simulink model "Mpc_RealTime_with_standing"  (R2017b)
settings: Solver=FixedStepDiscrete  StartTime=0.0  StopTime=inf  FixedStep=0.0005  RelTol=1e-3  EnableMultiTasking=on
InitFcn:
  | isSim = 0;
  | PreFunctions.CustomInitFcn_with_standing;
undefined symbols (not defined in the file): DynamicMatrixLibrary, sample_time
libraries: slrtlib x29, xpcrtudplib x2, xpcutilitieslib x1, CassieLibrary x1
settings Model: xpc_rtwmakecfg_data=_xpcethercatlib_  TunableVars=c_CovPos_abduction,c_CovPos_knee,c_CovPos_qj1,c_CovPos_qj2,c_CovPos_qj3,c_CovPos_rotation,c_CovPos_thigh,c_CovPos_toe,c_CovVel_abduction,c_CovVel_knee,c_CovVel_qj1,c_CovVel_qj2,c_CovVel_qj3,c_CovVel_rotation,c_CovVel_thigh,c_CovVel_toe,c_Cov_AngularVelocity,c_Cov_Euler,c_Cov_Euler_rates,c_Cov_LinearAccelerator_xy,c_Cov_LinearAccelerator_z,c_Cov_Lx_LRToe_stTD0,c_Cov_Ly_LRToe_stTD0,c_Cov_Orientation,c_Cov_rpx_LRToe_body,c_Cov_rpx_LRToe_stTD0,c_Cov_rpy_LRToe_body,c_Cov_rpy_LRToe_stTD0,c_Cov_rpz_LRToe_body,c_H_fil_param,c_IK_max_iter_num,c_Kd_abduction,c_Kd_knee,c_Kd_pitch,c_Kd_roll,c_Kd_rotation,c_Kd_st_rotation,c_Kd_thigh,c_Kd_toe,c_Kd_yaw,c_Kp_abduction,c_Kp_knee,c_Kp_pitch,c_Kp_roll,c_Kp_rotation,c_Kp_st_rotation,c_Kp_thigh,c_Kp_toe,c_Kp_yaw,c_KsL_1,c_KsL_2,c_KsR_1,c_KsR_2,c_Tx_slide_toe_2,c_Ty_slide_toe_2,c_Tz_slide_toe_2,c_Vx_tgd_fil_param,c_Vx_tgd_offset,c_Vy_tgd_avg_fil_param,c_Vy_tgd_offset,c_adjusted_desired_roll_angle_fil_param,c_com_x_offset,c_desired_com2stToe_lateral_fil_param,c_dop,c_history_length,c_knee_cp_time,c_lateral_correction_gain,c_max_st_rotation_motor_torque,c_max_turn_per_sec,c_one_step_max_vel_gain,c_rp_LRToe_fil_param,c_st_rotation_torque_ramp_time,c_stance_thre_lb,c_stance_thre_lb_2,c_stance_thre_ub,c_stance_thre_ub_2,c_toe_leave_ground_lb,c_toe_leave_ground_ub,c_torque_transition_time,c_u_abduction_swing_cp,c_u_knee_cp,c_u_pitch_cp,c_u_roll_cp,c_use_dq_AR_for_PD,c_vx_slide_toe_1,c_vx_slide_toe_2,c_vy_slide_toe_1,c_vy_slide_toe_2,c_vz_slide_toe_1,c_vz_slide_toe_2,c_yaw_error_fil_param  TunableVarsStorageClass=Auto,Auto,Auto,Auto,Auto,Auto,Auto,Auto,Auto,Auto,Auto,Auto,Auto,Auto,Auto,Auto,Auto,Auto,Auto,Auto,Auto,Auto,Auto,Auto,Auto,Auto,Auto,Auto,Auto,Auto,Auto,Auto,Auto,Auto,Auto,Auto,Auto,Auto,Auto,Auto,Auto,Auto,Auto,Auto,Auto,Auto,Auto,Auto,Auto,Auto,Auto,Auto,Auto,Auto,Auto,Auto,Auto,Auto,Auto,Auto,Auto,Auto,Auto,Auto,Auto,Auto,Auto,Auto,Auto,Auto,Auto,Auto,Auto,Auto,Auto,Auto,Auto,Auto,Auto,Auto,Auto,Auto,Auto,Auto,Auto,Auto,Auto,Auto,Auto,Auto,Auto  TunableVarsTypeQualifier=,,,,,,,,,,,,,,,,,,,,,,,,,,,,,,,,,,,,,,,,,,,,,,,,,,,,,,,,,,,,,,,,,,,,,,,,,,,,,,,,,,,,,,,,,,  Creator=robot  LastModifiedBy=gibso
settings DataIOCC: SaveFormat=Array  SaveOutput=off  SignalLogging=off  DSMLogging=off  VisualizeSimOutput=off  SaveTime=off
settings OptimizationCC: LifeSpan=inf  SimCompilerOptimization=on  AccelVerboseBuild=on
settings DebuggingCC: AllowSymbolicDim=off  SFUnexpectedBacktrackingDiag=warning  SFNoUnconditionalDefaultTransitionDiag=warning  SFExecutionAtInitializationDiag=none
settings HardwareCC: ProdBitPerPointer=32  ProdBitPerSizeT=32  ProdBitPerPtrDiffT=32  ProdLargestAtomicFloat=None  ProdWordSize=32  ProdLongLongMode=on  ProdHWDeviceType=Generic->32-bit x86 compatible
settings ModelReferenceCC: ParallelModelReferenceMATLABWorkerInit=Copy Base Workspace  ModelReferenceNumInstancesAllowed=Zero  PropagateSignalLabelsOutOfModel=off
settings SFSimCC: SimUserIncludeDirs=C:\Users\gibso\workspace\research\cassie_mpc_lip\matlab\Custom_Code\utils\funcs\KinDyn200511_221619  SFSimEcho=off
settings SFSimCC: SimUserSources=|
  | R_LeftAbductionJoint_src.c
  | R_LeftThighJoint_src.c
  | R_RightAbductionJoint_src.c
  | R_RightThighJoint_src.c
  | 
  | AMworld_about_pA_src.c
  | 
  | Jb_BasePosX_src.c
  | Jb_BasePosY_src.c
  | Jb_BasePosZ_src.c
  | Jb_BaseRotX_src.c
  | Jb_BaseRotY_src.c
  | Jb_BaseRotZ_src.c
  | Jb_LeftAbductionJoint_src.c
  | Jb_LeftAnkleJoint_src.c
  | Jb_LeftHip_src.c
  | Jb_LeftKneeJoint_src.c
  | Jb_LeftKneeSpringJoint_src.c
  | Jb_LeftKnee_src.c
  | Jb_LeftPelvisRotation_src.c
  | Jb_LeftRotationJoint_src.c
  | Jb_LeftShin_src.c
  | Jb_LeftTarsus_src.c
  | Jb_LeftThighJoint_src.c
  | Jb_LeftThigh_src.c
  | Jb_LeftToeBottomBack_src.c
  | Jb_LeftToeBottomFront_src.c
  | Jb_LeftToeBottom_src.c
  | Jb_LeftToeJoint_src.c
  | Jb_LeftToe_src.c
  | Jb_Pelvis_src.c
  | Jb_RightAbductionJoint_src.c
  | Jb_RightAnkleJoint_src.c
  | Jb_RightHip_src.c
  | Jb_RightKneeJoint_src.c
  | Jb_RightKneeSpringJoint_src.c
  | Jb_RightKnee_src.c
  | Jb_RightPelvisRotation_src.c
  | Jb_RightRotationJoint_src.c
  | Jb_RightShin_src.c
  | Jb_RightTarsus_src.c
  | Jb_RightThighJoint_src.c
  | Jb_RightThigh_src.c
  | Jb_RightToeBottomBack_src.c
  | Jb_RightToeBottomFront_src.c
  | Jb_RightToeBottom_src.c
  | Jb_RightToeJoint_src.c
  | Jb_RightToe_src.c
  | 
  | Jdq_AMworld_about_pA_src.c
  | 
  | 
  | Jp_COM_src.c
  | Jp_LeftAbductionJoint_src.c
  | Jp_LeftAnkleJoint_src.c
  | Jp_LeftHip_src.c
  | Jp_LeftKneeJoint_src.c
  | Jp_LeftKneeSpringJoint_src.c
  | Jp_LeftKnee_src.c
  | Jp_LeftPelvisRotation_src.c
  | Jp_LeftRotationJoint_src.c
  | Jp_LeftShin_src.c
  | Jp_LeftTarsus_src.c
  | Jp_LeftThighJoint_src.c
  | Jp_LeftThigh_src.c
  | Jp_LeftToeBottomBack_src.c
  | Jp_LeftToeBottomFront_src.c
  | Jp_LeftToeBottom_src.c
  | Jp_LeftToeJoint_src.c
  | Jp_LeftToe_src.c
  | Jp_Pelvis_src.c
  | Jp_RightAbductionJoint_src.c
  | Jp_RightAnkleJoint_src.c
  | Jp_RightHip_src.c
  | Jp_RightKneeJoint_src.c
  | Jp_RightKneeSpringJoint_src.c
  | Jp_RightKnee_src.c
  | Jp_RightPelvisRotation_src.c
  | Jp_RightRotationJoint_src.c
  | Jp_RightShin_src.c
  | Jp_RightTarsus_src.c
  | Jp_RightThighJoint_src.c
  | Jp_RightThigh_src.c
  | Jp_RightToeBottomBack_src.c
  | Jp_RightToeBottomFront_src.c
  | Jp_RightToeBottom_src.c
  | Jp_RightToeJoint_src.c
  | Jp_RightToe_src.c
  | 
  | p_BasePosX_src.c
  | p_BasePosY_src.c
  | p_BasePosZ_src.c
  | p_BaseRotX_src.c
  | p_BaseRotY_src.c
  | p_BaseRotZ_src.c
  | p_COM_src.c
  | p_LeftAbductionJoint_src.c
  | p_LeftAnkleJoint_src.c
  | p_LeftHip_src.c
  | p_LeftKneeJoint_src.c
  | p_LeftKneeSpringJoint_src.c
  | p_LeftKnee_src.c
  | p_LeftPelvisRotation_src.c
  | p_LeftRotationJoint_src.c
  | p_LeftShin_src.c
  | p_LeftTarsus_src.c
  | p_LeftThighJoint_src.c
  | p_LeftThigh_src.c
  | p_LeftToeBottomBack_src.c
  | p_LeftToeBottomFront_src.c
  | p_LeftToeBottom_src.c
  | p_LeftToeJoint_src.c
  | p_LeftToe_src.c
  | p_Pelvis_src.c
  | p_RightAbductionJoint_src.c
  | p_RightAnkleJoint_src.c
  | p_RightHip_src.c
  | p_RightKneeJoint_src.c
  | p_RightKneeSpringJoint_src.c
  | p_RightKnee_src.c
  | p_RightPelvisRotation_src.c
  | p_RightRotationJoint_src.c
  | p_RightShin_src.c
  | p_RightTarsus_src.c
  | p_RightThighJoint_src.c
  | p_RightThigh_src.c
  | p_RightToeBottomBack_src.c
  | p_RightToeBottomFront_src.c
  | p_RightToeBottom_src.c
  | p_RightToeJoint_src.c
  | p_RightToe_src.c
  | 
  | T_LeftToeBottomBack_src.c
  | T_LeftToeBottomFront_src.c
  | T_LeftToeBottom_src.c
  | T_RightToeBottomBack_src.c
  | T_RightToeBottomFront_src.c
  | T_RightToeBottom_src.c
  | 
  | J_LL_Left_src.c
  | J_LL_Right_src.c
  | LL_Left_src.c
  | LL_Right_src.c
settings RTWCC: SystemTargetFile=slrt.tlc  TLCOptions=-axPCMaxOverloads=1000000000 -axPCMaxOverloadLen=1000000000  TemplateMakefile=slrt_default_tmf  Description=Simulink Real-Time  RTWUseSimCustomCode=on  CustomInclude=C:\Users\gibso\workspace\research\cassie_mpc_lip\matlab\Custom_Code\utils\funcs\KinDyn200511_221619  CodeExecutionProfiling=on  RTWCompilerOptimization=on
settings RTWCC: CustomSource=|
  | R_LeftAbductionJoint_src.c
  | R_LeftThighJoint_src.c
  | R_RightAbductionJoint_src.c
  | R_RightThighJoint_src.c
  | 
  | AMworld_about_pA_src.c
  | 
  | Jb_BasePosX_src.c
  | Jb_BasePosY_src.c
  | Jb_BasePosZ_src.c
  | Jb_BaseRotX_src.c
  | Jb_BaseRotY_src.c
  | Jb_BaseRotZ_src.c
  | Jb_LeftAbductionJoint_src.c
  | Jb_LeftAnkleJoint_src.c
  | Jb_LeftHip_src.c
  | Jb_LeftKneeJoint_src.c
  | Jb_LeftKneeSpringJoint_src.c
  | Jb_LeftKnee_src.c
  | Jb_LeftPelvisRotation_src.c
  | Jb_LeftRotationJoint_src.c
  | Jb_LeftShin_src.c
  | Jb_LeftTarsus_src.c
  | Jb_LeftThighJoint_src.c
  | Jb_LeftThigh_src.c
  | Jb_LeftToeBottomBack_src.c
  | Jb_LeftToeBottomFront_src.c
  | Jb_LeftToeBottom_src.c
  | Jb_LeftToeJoint_src.c
  | Jb_LeftToe_src.c
  | Jb_Pelvis_src.c
  | Jb_RightAbductionJoint_src.c
  | Jb_RightAnkleJoint_src.c
  | Jb_RightHip_src.c
  | Jb_RightKneeJoint_src.c
  | Jb_RightKneeSpringJoint_src.c
  | Jb_RightKnee_src.c
  | Jb_RightPelvisRotation_src.c
  | Jb_RightRotationJoint_src.c
  | Jb_RightShin_src.c
  | Jb_RightTarsus_src.c
  | Jb_RightThighJoint_src.c
  | Jb_RightThigh_src.c
  | Jb_RightToeBottomBack_src.c
  | Jb_RightToeBottomFront_src.c
  | Jb_RightToeBottom_src.c
  | Jb_RightToeJoint_src.c
  | Jb_RightToe_src.c
  | 
  | Jdq_AMworld_about_pA_src.c
  | 
  | 
  | Jp_COM_src.c
  | Jp_LeftAbductionJoint_src.c
  | Jp_LeftAnkleJoint_src.c
  | Jp_LeftHip_src.c
  | Jp_LeftKneeJoint_src.c
  | Jp_LeftKneeSpringJoint_src.c
  | Jp_LeftKnee_src.c
  | Jp_LeftPelvisRotation_src.c
  | Jp_LeftRotationJoint_src.c
  | Jp_LeftShin_src.c
  | Jp_LeftTarsus_src.c
  | Jp_LeftThighJoint_src.c
  | Jp_LeftThigh_src.c
  | Jp_LeftToeBottomBack_src.c
  | Jp_LeftToeBottomFront_src.c
  | Jp_LeftToeBottom_src.c
  | Jp_LeftToeJoint_src.c
  | Jp_LeftToe_src.c
  | Jp_Pelvis_src.c
  | Jp_RightAbductionJoint_src.c
  | Jp_RightAnkleJoint_src.c
  | Jp_RightHip_src.c
  | Jp_RightKneeJoint_src.c
  | Jp_RightKneeSpringJoint_src.c
  | Jp_RightKnee_src.c
  | Jp_RightPelvisRotation_src.c
  | Jp_RightRotationJoint_src.c
  | Jp_RightShin_src.c
  | Jp_RightTarsus_src.c
  | Jp_RightThighJoint_src.c
  | Jp_RightThigh_src.c
  | Jp_RightToeBottomBack_src.c
  | Jp_RightToeBottomFront_src.c
  | Jp_RightToeBottom_src.c
  | Jp_RightToeJoint_src.c
  | Jp_RightToe_src.c
  | 
  | p_BasePosX_src.c
  | p_BasePosY_src.c
  | p_BasePosZ_src.c
  | p_BaseRotX_src.c
  | p_BaseRotY_src.c
  | p_BaseRotZ_src.c
  | p_COM_src.c
  | p_LeftAbductionJoint_src.c
  | p_LeftAnkleJoint_src.c
  | p_LeftHip_src.c
  | p_LeftKneeJoint_src.c
  | p_LeftKneeSpringJoint_src.c
  | p_LeftKnee_src.c
  | p_LeftPelvisRotation_src.c
  | p_LeftRotationJoint_src.c
  | p_LeftShin_src.c
  | p_LeftTarsus_src.c
  | p_LeftThighJoint_src.c
  | p_LeftThigh_src.c
  | p_LeftToeBottomBack_src.c
  | p_LeftToeBottomFront_src.c
  | p_LeftToeBottom_src.c
  | p_LeftToeJoint_src.c
  | p_LeftToe_src.c
  | p_Pelvis_src.c
  | p_RightAbductionJoint_src.c
  | p_RightAnkleJoint_src.c
  | p_RightHip_src.c
  | p_RightKneeJoint_src.c
  | p_RightKneeSpringJoint_src.c
  | p_RightKnee_src.c
  | p_RightPelvisRotation_src.c
  | p_RightRotationJoint_src.c
  | p_RightShin_src.c
  | p_RightTarsus_src.c
  | p_RightThighJoint_src.c
  | p_RightThigh_src.c
  | p_RightToeBottomBack_src.c
  | p_RightToeBottomFront_src.c
  | p_RightToeBottom_src.c
  | p_RightToeJoint_src.c
  | p_RightToe_src.c
  | 
  | T_LeftToeBottomBack_src.c
  | T_LeftToeBottomFront_src.c
  | T_LeftToeBottom_src.c
  | T_RightToeBottomBack_src.c
  | T_RightToeBottomFront_src.c
  | T_RightToeBottom_src.c
  | 
  | J_LL_Left_src.c
  | J_LL_Right_src.c
  | LL_Left_src.c
  | LL_Right_src.c
settings CodeAppCC: GenerateComments=off  MaxIdLength=128  SimulinkBlockComments=off
settings ConfigComp: CovMetricSettings=dw  CovHtmlReporting=on  CovSaveCumulativeToWorkspaceVar=on  CovSaveSingleToWorkspaceVar=on  CovExternalEMLEnable=off

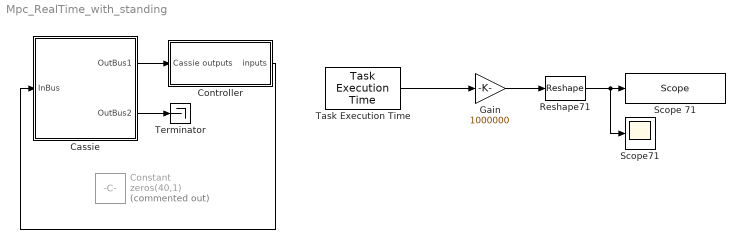
== system Mpc_RealTime_with_standing ==
  Cassie : Subsystem  AncestorBlock=CassieLibrary/RealTime/Cassie  InitFcn=|
      | % Import bus definitions
      | CassieModule.importBuses;
      mask Display: image('Cassie.png');
  Constant : Constant  Commented=on  Value=zeros(40,1)
  Controller : Subsystem
  Gain : Gain  Gain=1000000
  Reshape71 : Reshape
  Scope 71 : slrtlib/Displays and Logging/Scope   scopeno=1234  scopetype=Host  autostart=on  viewmode=Graphical redraw  formatstr='%15.6f'  grid=on  ylimits=[0,0]  nosamples=2500  noprepostsamples=0  interleave=1  triggermode=FreeRun  triggersignal=1  trigsignalfromport=off  triggerlevel=0.0  triggerslope=Either  triggerscope=1  triggersample=0  filename=data.dat  mode=Lazy  writesize=512  autorestart=off  dynamicfilemode=off  maxwritefilesize=512*1024^2
  Scope71 : Scope
  "Task Execution Time " : slrtlib/Target Management/Execution Parameters/Task Execution Time   ts=0.0005
      settings: SourceProductName=Simulink Real-Time  SourceProductBaseCode=XP
  Terminator : Terminator
  wires:
  Controller/1("inputs ") -> Cassie/1(InBus)
  Cassie/1(OutBus1) -> Controller/1(Cassie outputs)
  Reshape71/1 -> Scope71/1, Scope 71/1
  "Task Execution Time "/1 -> Gain/1
  Gain/1 -> Reshape71/1
  Cassie/2(OutBus2) -> Terminator/1

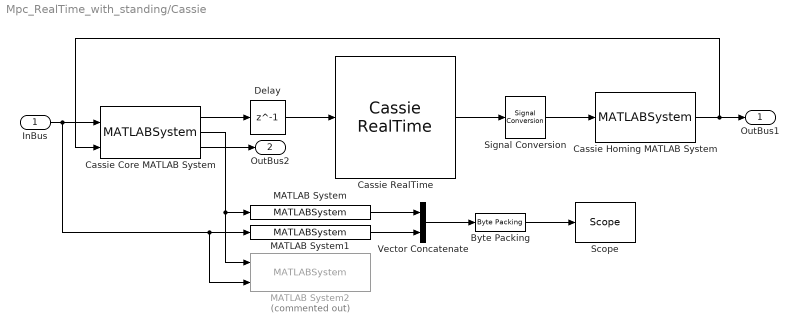
== system Mpc_RealTime_with_standing/Cassie ==
  InBus : Inport  OutDataTypeStr=Bus: CassieUserInBus
  "Byte Packing " : xpcutilitieslib/Byte Packing   MaskPackedDataType=double  MaskUnpackedDataTypes={'uint8'}  MaskAlignment=1
  Cassie Core MATLAB System : MATLABSystem  System=CassieCore  SimulateUsing=Code generation
      mask Type: CassieCore
      mask Display: disp('CassieCore');
  Cassie Homing MATLAB System : MATLABSystem  System=CassieHoming  SimulateUsing=Code generation
      mask Type: CassieHoming
      mask Display: disp('CassieHoming');
  Cassie RealTime : CassieLibrary/RealTime/Cassie RealTime  SystemSampleTime=-1
  Delay : Delay  DelayLength=1
  MATLAB System : MATLABSystem  System=CassieOutBusToBytes  SimulateUsing=Code generation
      mask Type: CassieOutBusToBytes
      mask Display: disp('CassieOutBusToBytes');
  MATLAB System1 : MATLABSystem  System=CassieUserInBusToBytes  SimulateUsing=Code generation
      mask Type: CassieUserInBusToBytes
      mask Display: disp('CassieUserInBusToBytes');
  MATLAB System2 : MATLABSystem  Commented=on  System=CassieSummaryLogger  period=1000  SimulateUsing=Code generation
      mask Type: CassieSummaryLogger
      mask Display: disp('CassieSummaryLogger');
  "Scope " : slrtlib/Displays and Logging/Scope   scopeno=1  scopetype=File  autostart=on  viewmode=Graphical redraw  formatstr='%15.6f'  grid=on  ylimits=[0,0]  nosamples=250  noprepostsamples=0  interleave=1  triggermode=FreeRun  triggersignal=1  trigsignalfromport=off  triggerlevel=0.0  triggerslope=Either  triggerscope=1  triggersample=0  filename=cassie<%%>.dat  mode=Commit  writesize=4096  autorestart=on  dynamicfilemode=on  maxwritefilesize=1024^3
  Signal Conversion : SignalConversion  ConversionOutput=Nonvirtual bus  OutDataTypeStr=Bus: CassieOutBus  OverrideOpt=off
  Vector Concatenate : Concatenate
  OutBus1 : Outport  OutDataTypeStr=Bus: CassieOutBus
  OutBus2 : Outport  Port=2  OutDataTypeStr=boolean
  wires:
  Cassie Core MATLAB System/3 -> OutBus2/1
  Cassie Core MATLAB System/2 -> MATLAB System/1, MATLAB System2/1
  "Byte Packing "/1 -> "Scope "/1
  MATLAB System1/1 -> Vector Concatenate/2
  Vector Concatenate/1 -> "Byte Packing "/1
  MATLAB System/1 -> Vector Concatenate/1
  Cassie Homing MATLAB System/1 -> OutBus1/1, Cassie Core MATLAB System/2
  Signal Conversion/1 -> Cassie Homing MATLAB System/1
  Delay/1 -> Cassie RealTime/1
  Cassie Core MATLAB System/1 -> Delay/1
  InBus/1 -> MATLAB System1/1, MATLAB System2/2, Cassie Core MATLAB System/1
  Cassie RealTime/1 -> Signal Conversion/1

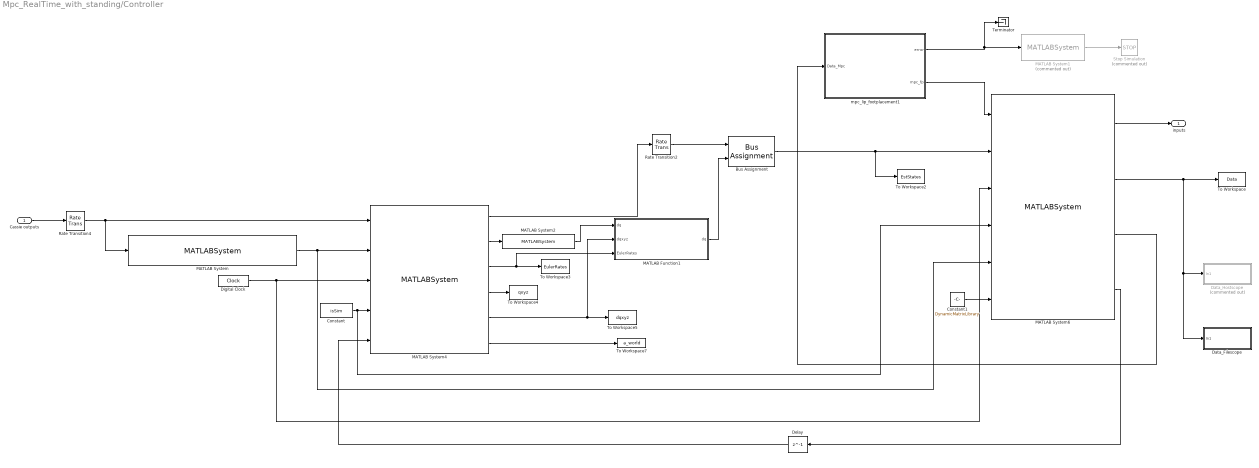
== system Mpc_RealTime_with_standing/Controller ==
  Cassie outputs : Inport  OutDataTypeStr=Bus: CassieOutBus
  Bus Assignment : BusAssignment  AssignedSignals=dq
  Constant : Constant  Value=isSim  OutDataTypeStr=int8  LockScale=on
  Constant1 : Constant  Value=DynamicMatrixLibrary  OutDataTypeStr=Bus: cassieDynamicMatrixLibraryBus
  Data_Filescope : Subsystem
  Data_Hostscope : Subsystem  Commented=on
  Delay : Delay  DelayLength=1  InitialCondition=0
  Digital Clock : DigitalClock  SampleTime=sample_time
  MATLAB Function1 : MATLAB Function  TreatAsAtomicUnit=on
  MATLAB System : MATLABSystem  System=RadioCommandInterpreter_with_standing  max_turn_per_sec=c_max_turn_per_sec  Vx_tgd_fil_param=c_Vx_tgd_fil_param  Vy_tgd_avg_fil_param=c_Vy_tgd_avg_fil_param  H_fil_param=c_H_fil_param  desired_com2stToe_lateral_fil_param=c_desired_com2stToe_lateral_fil_param  yaw_stand_filter_param=c_yaw_stand_filter_param  pitch_stand_filter_param=c_pitch_stand_filter_param  roll_stand_filter_param=c_roll_stand_filter_param  p_com_stand_y_filter_param=c_p_com_stand_y_filter_param  sample_time=sample_time  SimulateUsing=Code generation
      mask Type: RadioCommandInterpreter_with_standing
      mask Display:
      | disp('RadioCommandInterpreter_with_standing');
      | port_label('input',1,'cassieOutputs');
      | port_label('output',1,'IRC');
  MATLAB System1 : MATLABSystem  Commented=on  System=Error_Checker  SimulateUsing=Code generation
      mask Type: Error_Checker
      mask Display:
      | disp('Error_Checker');
      | port_label('input',1,'u');
      | port_label('output',1,'y');
  MATLAB System2 : MATLABSystem  System=PolyRegressionFilter_2  sample_time=sample_time  history_length=c_history_length  dop=c_dop  signal_dim=20  delay=0  max_history_length=20  max_dop=3  SimulateUsing=Code generation
      mask Type: PolyRegressionFilter_2
      mask Display:
      | disp('PolyRegressionFilter_2');
      | port_label('input',1,'q');
      | port_label('output',1,'dq');
  MATLAB System4 : MATLABSystem  System=StateEstimator_with_standing  Ks_L1=c_KsL_1  Ks_L2=c_KsL_2  Ks_R1=c_KsR_1  Ks_R2=c_KsR_2  Cov_LRT_r_body_x=c_Cov_rpx_LRToe_body  Cov_LRT_r_body_y=c_Cov_rpy_LRToe_body  Cov_LRT_r_body_z=c_Cov_rpz_LRToe_body  Cov_LinearAccelerator_xy=c_Cov_LinearAccelerator_xy  Cov_LinearAccelerator_z=c_Cov_LinearAccelerator_z  vx_slide_toe_1=c_vx_slide_toe_1  vx_slide_toe_2=c_vx_slide_toe_2  Tx_slide_toe_2=c_Tx_slide_toe_2  vy_slide_toe_1=c_vy_slide_toe_1  vy_slide_toe_2=c_vy_slide_toe_2  Ty_slide_toe_2=c_Ty_slide_toe_2  vz_slide_toe_1=c_vz_slide_toe_1  vz_slide_toe_2=c_vz_slide_toe_2  Tz_slide_toe_2=c_Tz_slide_toe_2  sample_time=sample_time  SimulateUsing=Code generation
      mask Type: StateEstimator_with_standing
      mask Display:
      | disp('StateEstimator_with_standing');
      | port_label('input',1,'cassieOutputs');
      | port_label('input',2,'IRC');
      | port_label('input',3,'t_total');
      | port_label('input',4,'isSim');
      | port_label('input',5,'Controller2Estimator');
      | port_label('output',1,'EstStates');
      | port_label('output',2,'q');
      | port_label('output',3,'EulerRates');
      | port_label('output',4,'q_xyz');
      | port_label('output',5,'dq_xyz');
      | port_label('output',6,'a_world');
  MATLAB System6 : MATLABSystem  System=Cassie_MPC_With_Standing  Kp_pitch=c_Kp_pitch  Kd_pitch=c_Kd_pitch  Kp_roll=c_Kp_roll  Kd_roll=c_Kd_roll  Kp_yaw=c_Kp_yaw  Kd_yaw=c_Kd_yaw  Kp_abduction=c_Kp_abduction  Kp_rotation=c_Kp_rotation  Kp_thigh=c_Kp_thigh  Kp_knee=c_Kp_knee  Kp_toe=c_Kp_toe  Kd_abduction=c_Kd_abduction  Kd_rotation=c_Kd_rotation  Kd_thigh=c_Kd_thigh  Kd_knee=c_Kd_knee  Kd_toe=c_Kd_toe  Kp_st_rotation=c_Kp_st_rotation  Kd_st_rotation=c_Kd_st_rotation  u_abduction_swing_cp=c_u_abduction_swing_cp  u_roll_cp=c_u_roll_cp  u_pitch_cp=c_u_pitch_cp  u_knee_cp=c_u_knee_cp  CovPos_abduction=c_CovPos_abduction  CovPos_rotation=c_CovPos_rotation  CovPos_thigh=c_CovPos_thigh  CovPos_knee=c_CovPos_knee  CovPos_toe=c_CovPos_toe  CovPos_qj1=c_CovPos_qj1  CovPos_qj2=c_CovPos_qj2  CovPos_qj3=c_CovPos_qj3  CovVel_abduction=c_CovVel_abduction  CovVel_rotation=c_CovVel_rotation  CovVel_thigh=c_CovVel_thigh  CovVel_knee=c_CovVel_knee  CovVel_toe=c_CovVel_toe  CovVel_qj1=c_CovVel_qj1  CovVel_qj2=c_CovVel_qj2  CovVel_qj3=c_CovVel_qj3  Cov_Euler=c_Cov_Euler  Cov_Euler_rates=c_Cov_Euler_rates  Cov_Lx_LRToe_stTD0=c_Cov_Lx_LRToe_stTD0  Cov_Ly_LRToe_stTD0=c_Cov_Ly_LRToe_stTD0  Cov_rpx_LRToe_stTD0=c_Cov_rpx_LRToe_stTD0  Cov_rpy_LRToe_stTD0=c_Cov_rpy_LRToe_stTD0  torque_transition_time=c_torque_transition_time  knee_cp_time=c_knee_cp_time  st_rotation_torque_ramp_time=c_st_rotation_torque_ramp_time  torque_standFromWalk_transition_time=c_torque_standFromWalk_transition_time  com_x_offset=c_com_x_offset  Vx_tgd_offset=c_Vx_tgd_offset  Vy_tgd_offset=c_Vy_tgd_offset  stance_thre_lb=c_stance_thre_lb  stance_thre_ub=c_stance_thre_ub  stance_thre_lb_2=c_stance_thre_lb_2  stance_thre_ub_2=c_stance_thre_ub_2  IK_max_iter_num=c_IK_max_iter_num  yaw_error_fil_param=c_yaw_error_fil_param  rp_LRToe_fil_param=c_rp_LRToe_fil_param  adjusted_desired_roll_angle_fil_param=c_adjusted_desired_roll_angle_fil_param  use_dq_AR_for_PD=c_use_dq_AR_for_PD  lateral_correction_gain=c_lateral_correction_gain  one_step_max_vel_gain=c_one_step_max_vel_gain  max_st_rotation_motor_torque=c_max_st_rotation_motor_torque  KsL_1=c_KsL_1  KsL_2=c_KsL_2  KsR_1=c_KsR_1  KsR_2=c_KsR_2  toe_leave_ground_lb=c_toe_leave_ground_lb  toe_leave_ground_ub=c_toe_leave_ground_ub  Kp_abduction_stand=c_Kp_abduction_stand  Kp_rotation_stand=c_Kp_rotation_stand  Kp_thigh_stand=c_Kp_thigh_stand  Kp_knee_stand=c_Kp_knee_stand  Kp_toe_stand=c_Kp_toe_stand  Kd_abduction_stand=c_Kd_abduction_stand  Kd_rotation_stand=c_Kd_rotation_stand  Kd_thigh_stand=c_Kd_thigh_stand  Kd_knee_stand=c_Kd_knee_stand  Kd_toe_stand=c_Kd_toe_stand  Kp_knee_stand_lateral=c_Kp_knee_stand_lateral  Kd_knee_stand_lateral=c_Kd_knee_stand_lateral  com_x_offset_stand=c_com_x_offset_stand  F_st_lb_stand=c_F_st_lb_stand  F_st_ub_stand=c_F_st_ub_stand  com_y_offset_stand2walk=c_com_y_offset_stand2walk  last_width_walk2stand=c_last_width_walk2stand  V_com_x_offset_walk2stand=c_V_com_x_offset_walk2stand  mu_fil_param=c_mu_fil_param  sample_time=sample_time  SimulateUsing=Code generation
      mask Type: Cassie_MPC_With_Standing
      mask Display:
      | disp('Cassie_MPC_With_Standing');
      | port_label('input',1,'mpc_fp');
      | port_label('input',2,'Est_States_Bus');
      | port_label('input',3,'t_total');
      | port_label('input',4,'isSim');
      | port_label('input',5,'IRC');
      | port_label('input',6,'DynamicMatrixLibrary');
      | port_label('output',1,'userInputs');
      | port_label('output',2,'Data');
      | port_label('output',3,'CustomEstStates');
      | port_label('output',4,'Controller2Estimator');
  Rate Transition2 : RateTransition  OutPortSampleTime=sample_time
  Rate Transition4 : RateTransition  OutPortSampleTime=sample_time
  Stop Simulation : Stop  Commented=on
  Terminator : Terminator
  To Workspace : ToWorkspace  VariableName=Data  SaveFormat=Timeseries  SampleTime=-1
  To Workspace2 : ToWorkspace  VariableName=EstStates  SaveFormat=Timeseries  SampleTime=-1
  To Workspace3 : ToWorkspace  VariableName=EulerRates  SaveFormat=Timeseries  SampleTime=-1
  To Workspace4 : ToWorkspace  VariableName=qxyz  SaveFormat=Timeseries  SampleTime=-1
  To Workspace5 : ToWorkspace  VariableName=dqxyz  SaveFormat=Timeseries  SampleTime=-1
  To Workspace7 : ToWorkspace  VariableName=a_world  SaveFormat=Timeseries  SampleTime=-1
  mpc_lip_footplacement1 : Subsystem
  "inputs " : Outport
  wires:
  Delay/1 -> MATLAB System4/5
  MATLAB System6/4 -> Delay/1
  MATLAB System4/2 -> MATLAB System2/1
  MATLAB System4/3 -> To Workspace3/1, MATLAB Function1/3(EulerRates)
  MATLAB System4/5 -> MATLAB Function1/2(dqxyz), To Workspace5/1
  MATLAB System4/4 -> To Workspace4/1
  MATLAB System6/3 -> mpc_lip_footplacement1/1(Data_Mpc)
  mpc_lip_footplacement1/1(error) -> MATLAB System1/1, Terminator/1
  MATLAB System1/1 -> Stop Simulation/1
  mpc_lip_footplacement1/2(mpc_fp) -> MATLAB System6/1
  Bus Assignment/1 -> To Workspace2/1, MATLAB System6/2
  MATLAB System6/2 -> To Workspace/1, Data_Hostscope/1(In1), Data_Filescope/1(In1)
  Rate Transition2/1 -> Bus Assignment/1
  MATLAB System/1 -> MATLAB System4/2, MATLAB System6/5
  MATLAB System4/1 -> Rate Transition2/1
  MATLAB System2/1 -> MATLAB Function1/1("dq ")
  MATLAB Function1/1(dq) -> Bus Assignment/2
  Rate Transition4/1 -> MATLAB System4/1, MATLAB System/1
  MATLAB System6/1 -> "inputs "/1
  Constant1/1 -> MATLAB System6/6
  Cassie outputs/1 -> Rate Transition4/1
  Constant/1 -> MATLAB System4/4, MATLAB System6/4
  Digital Clock/1 -> MATLAB System4/3, MATLAB System6/3
  MATLAB System4/6 -> To Workspace7/1

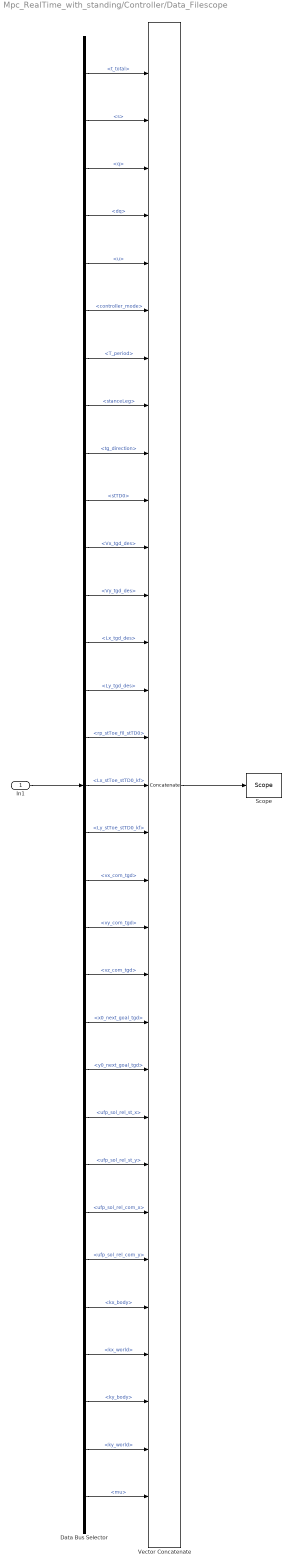
== system Mpc_RealTime_with_standing/Controller/Data_Filescope ==
  In1 : Inport  OutDataTypeStr=Bus: cassieDataWithStandingBus
  Data Bus Selector : BusSelector  OutputSignals=t_total,s,q,dq,u,controller_mode,T_period,stanceLeg,tg_direction,stTD0,Vx_tgd_des,Vy_tgd_des,Lx_tgd_des,Ly_tgd_des,rp_stToe_fil_stTD0,Lx_stToe_stTD0_kf,Ly_stToe_stTD0_kf,vx_com_tgd,vy_com_tgd,vz_com_tgd,x0_next_goal_tgd,y0_next_goal_tgd,ufp_sol_rel_st_x,ufp_sol_rel_st_y,ufp_sol_rel_com_x,ufp_sol_rel_com_y,kx_body,kx_world,ky_body,ky_world,mu
  "Scope " : slrtlib/Displays and Logging/Scope   scopeno=5  scopetype=File  autostart=on  viewmode=Graphical redraw  formatstr='%15.6f'  grid=on  ylimits=[0,0]  nosamples=250  noprepostsamples=0  interleave=1  triggermode=FreeRun  triggersignal=1  trigsignalfromport=off  triggerlevel=0.0  triggerslope=Either  triggerscope=1  triggersample=0  filename=DATA<%%>.dat  mode=Commit  writesize=4096  autorestart=on  dynamicfilemode=on  maxwritefilesize=1024^3
  Vector Concatenate : Concatenate  NumInputs=31
  wires:
  Vector Concatenate/1 -> "Scope "/1
  In1/1 -> Data Bus Selector/1
  Data Bus Selector/1 -> Vector Concatenate/1  "<t_total>"
  Data Bus Selector/2 -> Vector Concatenate/2  "<s>"
  Data Bus Selector/3 -> Vector Concatenate/3  "<q>"
  Data Bus Selector/4 -> Vector Concatenate/4  "<dq>"
  Data Bus Selector/5 -> Vector Concatenate/5  "<u>"
  Data Bus Selector/6 -> Vector Concatenate/6  "<controller_mode>"
  Data Bus Selector/7 -> Vector Concatenate/7  "<T_period>"
  Data Bus Selector/8 -> Vector Concatenate/8  "<stanceLeg>"
  Data Bus Selector/9 -> Vector Concatenate/9  "<tg_direction>"
  Data Bus Selector/10 -> Vector Concatenate/10  "<stTD0>"
  Data Bus Selector/11 -> Vector Concatenate/11  "<Vx_tgd_des>"
  Data Bus Selector/12 -> Vector Concatenate/12  "<Vy_tgd_des>"
  Data Bus Selector/13 -> Vector Concatenate/13  "<Lx_tgd_des>"
  Data Bus Selector/14 -> Vector Concatenate/14  "<Ly_tgd_des>"
  Data Bus Selector/15 -> Vector Concatenate/15  "<rp_stToe_fil_stTD0>"
  Data Bus Selector/16 -> Vector Concatenate/16  "<Lx_stToe_stTD0_kf>"
  Data Bus Selector/17 -> Vector Concatenate/17  "<Ly_stToe_stTD0_kf>"
  Data Bus Selector/18 -> Vector Concatenate/18  "<vx_com_tgd>"
  Data Bus Selector/19 -> Vector Concatenate/19  "<vy_com_tgd>"
  Data Bus Selector/20 -> Vector Concatenate/20  "<vz_com_tgd>"
  Data Bus Selector/21 -> Vector Concatenate/21  "<x0_next_goal_tgd>"
  Data Bus Selector/22 -> Vector Concatenate/22  "<y0_next_goal_tgd>"
  Data Bus Selector/23 -> Vector Concatenate/23  "<ufp_sol_rel_st_x>"
  Data Bus Selector/24 -> Vector Concatenate/24  "<ufp_sol_rel_st_y>"
  Data Bus Selector/25 -> Vector Concatenate/25  "<ufp_sol_rel_com_x>"
  Data Bus Selector/26 -> Vector Concatenate/26  "<ufp_sol_rel_com_y>"
  Data Bus Selector/27 -> Vector Concatenate/27  "<kx_body>"
  Data Bus Selector/28 -> Vector Concatenate/28  "<kx_world>"
  Data Bus Selector/29 -> Vector Concatenate/29  "<ky_body>"
  Data Bus Selector/30 -> Vector Concatenate/30  "<ky_world>"
  Data Bus Selector/31 -> Vector Concatenate/31  "<mu>"

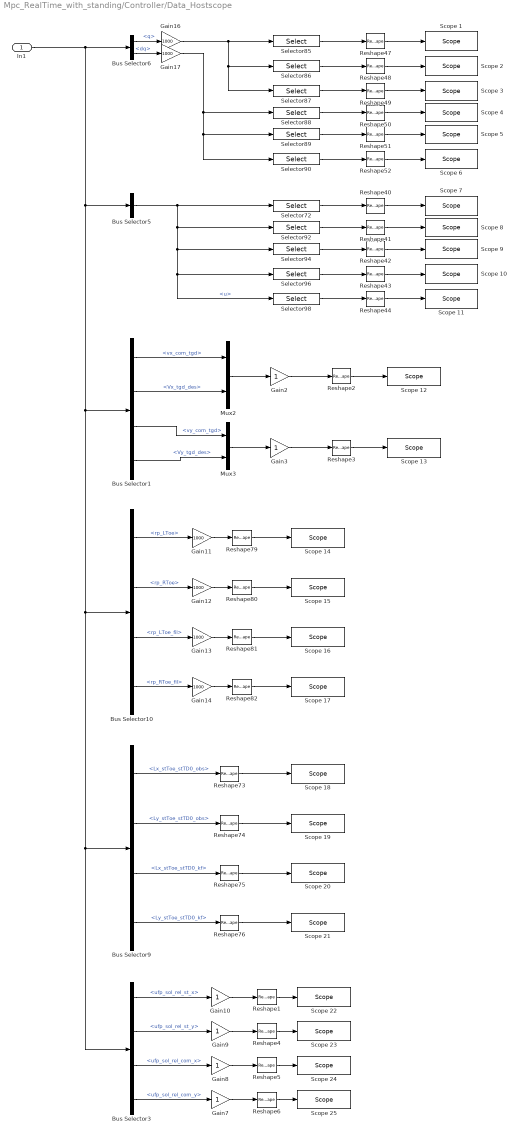
== system Mpc_RealTime_with_standing/Controller/Data_Hostscope ==
  In1 : Inport
  Bus Selector1 : BusSelector  OutputSignals=vx_com_tgd,Vx_tgd_des,vy_com_tgd,Vy_tgd_des
  Bus Selector10 : BusSelector  OutputSignals=rp_LToe,rp_RToe,rp_LToe_fil,rp_RToe_fil
  Bus Selector3 : BusSelector  OutputSignals=ufp_sol_rel_st_x,ufp_sol_rel_st_y,ufp_sol_rel_com_x,ufp_sol_rel_com_y
  Bus Selector5 : BusSelector  OutputSignals=u
  Bus Selector6 : BusSelector  OutputSignals=q,dq
  Bus Selector9 : BusSelector  OutputSignals=Lx_stToe_stTD0_obs,Ly_stToe_stTD0_obs,Lx_stToe_stTD0_kf,Ly_stToe_stTD0_kf
  Gain{2..3,7..10} (6 alike) : Gain
  Gain{11..14,16..17} (6 alike) : Gain  Gain=1000
  Mux2 : Mux  Inputs=2
  Mux3 : Mux  Inputs=2
  Reshape{1..6,40..44,47..52,73..76,79..82} (25 alike) : Reshape
  Scope 1 : slrtlib/Displays and Logging/Scope   scopeno=101  scopetype=Host  autostart=on  viewmode=Graphical redraw  formatstr='%15.6f'  grid=on  ylimits=[0,0]  nosamples=250  noprepostsamples=0  interleave=1  triggermode=FreeRun  triggersignal=1  trigsignalfromport=off  triggerlevel=0.0  triggerslope=Either  triggerscope=1  triggersample=0  filename=data.dat  mode=Lazy  writesize=512  autorestart=off  dynamicfilemode=off  maxwritefilesize=512*1024^2
  Scope 10 : slrtlib/Displays and Logging/Scope   scopeno=110  scopetype=Host  autostart=on  viewmode=Graphical redraw  formatstr='%15.6f'  grid=on  ylimits=[0,0]  nosamples=250  noprepostsamples=0  interleave=1  triggermode=FreeRun  triggersignal=1  trigsignalfromport=off  triggerlevel=0.0  triggerslope=Either  triggerscope=1  triggersample=0  filename=data.dat  mode=Lazy  writesize=512  autorestart=off  dynamicfilemode=off  maxwritefilesize=512*1024^2
  Scope 11 : slrtlib/Displays and Logging/Scope   scopeno=111  scopetype=Host  autostart=on  viewmode=Graphical redraw  formatstr='%15.6f'  grid=on  ylimits=[0,0]  nosamples=250  noprepostsamples=0  interleave=1  triggermode=FreeRun  triggersignal=1  trigsignalfromport=off  triggerlevel=0.0  triggerslope=Either  triggerscope=1  triggersample=0  filename=data.dat  mode=Lazy  writesize=512  autorestart=off  dynamicfilemode=off  maxwritefilesize=512*1024^2
  Scope 12 : slrtlib/Displays and Logging/Scope   scopeno=112  scopetype=Host  autostart=on  viewmode=Graphical redraw  formatstr='%15.6f'  grid=on  ylimits=[0,0]  nosamples=250  noprepostsamples=0  interleave=1  triggermode=FreeRun  triggersignal=1  trigsignalfromport=off  triggerlevel=0.0  triggerslope=Either  triggerscope=1  triggersample=0  filename=data.dat  mode=Lazy  writesize=512  autorestart=off  dynamicfilemode=off  maxwritefilesize=512*1024^2
  Scope 13 : slrtlib/Displays and Logging/Scope   scopeno=113  scopetype=Host  autostart=on  viewmode=Graphical redraw  formatstr='%15.6f'  grid=on  ylimits=[0,0]  nosamples=250  noprepostsamples=0  interleave=1  triggermode=FreeRun  triggersignal=1  trigsignalfromport=off  triggerlevel=0.0  triggerslope=Either  triggerscope=1  triggersample=0  filename=data.dat  mode=Lazy  writesize=512  autorestart=off  dynamicfilemode=off  maxwritefilesize=512*1024^2
  Scope 14 : slrtlib/Displays and Logging/Scope   scopeno=114  scopetype=Host  autostart=on  viewmode=Graphical redraw  formatstr='%15.6f'  grid=on  ylimits=[0,0]  nosamples=250  noprepostsamples=0  interleave=1  triggermode=FreeRun  triggersignal=1  trigsignalfromport=off  triggerlevel=0.0  triggerslope=Either  triggerscope=1  triggersample=0  filename=data.dat  mode=Lazy  writesize=512  autorestart=off  dynamicfilemode=off  maxwritefilesize=512*1024^2
  Scope 15 : slrtlib/Displays and Logging/Scope   scopeno=115  scopetype=Host  autostart=on  viewmode=Graphical redraw  formatstr='%15.6f'  grid=on  ylimits=[0,0]  nosamples=250  noprepostsamples=0  interleave=1  triggermode=FreeRun  triggersignal=1  trigsignalfromport=off  triggerlevel=0.0  triggerslope=Either  triggerscope=1  triggersample=0  filename=data.dat  mode=Lazy  writesize=512  autorestart=off  dynamicfilemode=off  maxwritefilesize=512*1024^2
  Scope 16 : slrtlib/Displays and Logging/Scope   scopeno=116  scopetype=Host  autostart=on  viewmode=Graphical redraw  formatstr='%15.6f'  grid=on  ylimits=[0,0]  nosamples=250  noprepostsamples=0  interleave=1  triggermode=FreeRun  triggersignal=1  trigsignalfromport=off  triggerlevel=0.0  triggerslope=Either  triggerscope=1  triggersample=0  filename=data.dat  mode=Lazy  writesize=512  autorestart=off  dynamicfilemode=off  maxwritefilesize=512*1024^2
  Scope 17 : slrtlib/Displays and Logging/Scope   scopeno=117  scopetype=Host  autostart=on  viewmode=Graphical redraw  formatstr='%15.6f'  grid=on  ylimits=[0,0]  nosamples=250  noprepostsamples=0  interleave=1  triggermode=FreeRun  triggersignal=1  trigsignalfromport=off  triggerlevel=0.0  triggerslope=Either  triggerscope=1  triggersample=0  filename=data.dat  mode=Lazy  writesize=512  autorestart=off  dynamicfilemode=off  maxwritefilesize=512*1024^2
  Scope 18 : slrtlib/Displays and Logging/Scope   scopeno=118  scopetype=Host  autostart=on  viewmode=Graphical redraw  formatstr='%15.6f'  grid=on  ylimits=[0,0]  nosamples=250  noprepostsamples=0  interleave=1  triggermode=FreeRun  triggersignal=1  trigsignalfromport=off  triggerlevel=0.0  triggerslope=Either  triggerscope=1  triggersample=0  filename=data.dat  mode=Lazy  writesize=512  autorestart=off  dynamicfilemode=off  maxwritefilesize=512*1024^2
  Scope 19 : slrtlib/Displays and Logging/Scope   scopeno=119  scopetype=Host  autostart=on  viewmode=Graphical redraw  formatstr='%15.6f'  grid=on  ylimits=[0,0]  nosamples=250  noprepostsamples=0  interleave=1  triggermode=FreeRun  triggersignal=1  trigsignalfromport=off  triggerlevel=0.0  triggerslope=Either  triggerscope=1  triggersample=0  filename=data.dat  mode=Lazy  writesize=512  autorestart=off  dynamicfilemode=off  maxwritefilesize=512*1024^2
  Scope 2 : slrtlib/Displays and Logging/Scope   scopeno=102  scopetype=Host  autostart=on  viewmode=Graphical redraw  formatstr='%15.6f'  grid=on  ylimits=[0,0]  nosamples=250  noprepostsamples=0  interleave=1  triggermode=FreeRun  triggersignal=1  trigsignalfromport=off  triggerlevel=0.0  triggerslope=Either  triggerscope=1  triggersample=0  filename=data.dat  mode=Lazy  writesize=512  autorestart=off  dynamicfilemode=off  maxwritefilesize=512*1024^2
  Scope 20 : slrtlib/Displays and Logging/Scope   scopeno=120  scopetype=Host  autostart=on  viewmode=Graphical redraw  formatstr='%15.6f'  grid=on  ylimits=[0,0]  nosamples=250  noprepostsamples=0  interleave=1  triggermode=FreeRun  triggersignal=1  trigsignalfromport=off  triggerlevel=0.0  triggerslope=Either  triggerscope=1  triggersample=0  filename=data.dat  mode=Lazy  writesize=512  autorestart=off  dynamicfilemode=off  maxwritefilesize=512*1024^2
  Scope 21 : slrtlib/Displays and Logging/Scope   scopeno=121  scopetype=Host  autostart=on  viewmode=Graphical redraw  formatstr='%15.6f'  grid=on  ylimits=[0,0]  nosamples=250  noprepostsamples=0  interleave=1  triggermode=FreeRun  triggersignal=1  trigsignalfromport=off  triggerlevel=0.0  triggerslope=Either  triggerscope=1  triggersample=0  filename=data.dat  mode=Lazy  writesize=512  autorestart=off  dynamicfilemode=off  maxwritefilesize=512*1024^2
  Scope 22 : slrtlib/Displays and Logging/Scope   scopeno=122  scopetype=Host  autostart=on  viewmode=Graphical redraw  formatstr='%15.6f'  grid=on  ylimits=[0,0]  nosamples=250  noprepostsamples=0  interleave=1  triggermode=FreeRun  triggersignal=1  trigsignalfromport=off  triggerlevel=0.0  triggerslope=Either  triggerscope=1  triggersample=0  filename=data.dat  mode=Lazy  writesize=512  autorestart=off  dynamicfilemode=off  maxwritefilesize=512*1024^2
  Scope 23 : slrtlib/Displays and Logging/Scope   scopeno=123  scopetype=Host  autostart=on  viewmode=Graphical redraw  formatstr='%15.6f'  grid=on  ylimits=[0,0]  nosamples=250  noprepostsamples=0  interleave=1  triggermode=FreeRun  triggersignal=1  trigsignalfromport=off  triggerlevel=0.0  triggerslope=Either  triggerscope=1  triggersample=0  filename=data.dat  mode=Lazy  writesize=512  autorestart=off  dynamicfilemode=off  maxwritefilesize=512*1024^2
  Scope 24 : slrtlib/Displays and Logging/Scope   scopeno=124  scopetype=Host  autostart=on  viewmode=Graphical redraw  formatstr='%15.6f'  grid=on  ylimits=[0,0]  nosamples=250  noprepostsamples=0  interleave=1  triggermode=FreeRun  triggersignal=1  trigsignalfromport=off  triggerlevel=0.0  triggerslope=Either  triggerscope=1  triggersample=0  filename=data.dat  mode=Lazy  writesize=512  autorestart=off  dynamicfilemode=off  maxwritefilesize=512*1024^2
  Scope 25 : slrtlib/Displays and Logging/Scope   scopeno=125  scopetype=Host  autostart=on  viewmode=Graphical redraw  formatstr='%15.6f'  grid=on  ylimits=[0,0]  nosamples=250  noprepostsamples=0  interleave=1  triggermode=FreeRun  triggersignal=1  trigsignalfromport=off  triggerlevel=0.0  triggerslope=Either  triggerscope=1  triggersample=0  filename=data.dat  mode=Lazy  writesize=512  autorestart=off  dynamicfilemode=off  maxwritefilesize=512*1024^2
  Scope 3 : slrtlib/Displays and Logging/Scope   scopeno=103  scopetype=Host  autostart=on  viewmode=Graphical redraw  formatstr='%15.6f'  grid=on  ylimits=[0,0]  nosamples=250  noprepostsamples=0  interleave=1  triggermode=FreeRun  triggersignal=1  trigsignalfromport=off  triggerlevel=0.0  triggerslope=Either  triggerscope=1  triggersample=0  filename=data.dat  mode=Lazy  writesize=512  autorestart=off  dynamicfilemode=off  maxwritefilesize=512*1024^2
  Scope 4 : slrtlib/Displays and Logging/Scope   scopeno=104  scopetype=Host  autostart=on  viewmode=Graphical redraw  formatstr='%15.6f'  grid=on  ylimits=[0,0]  nosamples=250  noprepostsamples=0  interleave=1  triggermode=FreeRun  triggersignal=1  trigsignalfromport=off  triggerlevel=0.0  triggerslope=Either  triggerscope=1  triggersample=0  filename=data.dat  mode=Lazy  writesize=512  autorestart=off  dynamicfilemode=off  maxwritefilesize=512*1024^2
  Scope 5 : slrtlib/Displays and Logging/Scope   scopeno=105  scopetype=Host  autostart=on  viewmode=Graphical redraw  formatstr='%15.6f'  grid=on  ylimits=[0,0]  nosamples=250  noprepostsamples=0  interleave=1  triggermode=FreeRun  triggersignal=1  trigsignalfromport=off  triggerlevel=0.0  triggerslope=Either  triggerscope=1  triggersample=0  filename=data.dat  mode=Lazy  writesize=512  autorestart=off  dynamicfilemode=off  maxwritefilesize=512*1024^2
  Scope 6 : slrtlib/Displays and Logging/Scope   scopeno=106  scopetype=Host  autostart=on  viewmode=Graphical redraw  formatstr='%15.6f'  grid=on  ylimits=[0,0]  nosamples=250  noprepostsamples=0  interleave=1  triggermode=FreeRun  triggersignal=1  trigsignalfromport=off  triggerlevel=0.0  triggerslope=Either  triggerscope=1  triggersample=0  filename=data.dat  mode=Lazy  writesize=512  autorestart=off  dynamicfilemode=off  maxwritefilesize=512*1024^2
  Scope 7 : slrtlib/Displays and Logging/Scope   scopeno=107  scopetype=Host  autostart=on  viewmode=Graphical redraw  formatstr='%15.6f'  grid=on  ylimits=[0,0]  nosamples=250  noprepostsamples=0  interleave=1  triggermode=FreeRun  triggersignal=1  trigsignalfromport=off  triggerlevel=0.0  triggerslope=Either  triggerscope=1  triggersample=0  filename=data.dat  mode=Lazy  writesize=512  autorestart=off  dynamicfilemode=off  maxwritefilesize=512*1024^2
  Scope 8 : slrtlib/Displays and Logging/Scope   scopeno=108  scopetype=Host  autostart=on  viewmode=Graphical redraw  formatstr='%15.6f'  grid=on  ylimits=[0,0]  nosamples=250  noprepostsamples=0  interleave=1  triggermode=FreeRun  triggersignal=1  trigsignalfromport=off  triggerlevel=0.0  triggerslope=Either  triggerscope=1  triggersample=0  filename=data.dat  mode=Lazy  writesize=512  autorestart=off  dynamicfilemode=off  maxwritefilesize=512*1024^2
  Scope 9 : slrtlib/Displays and Logging/Scope   scopeno=109  scopetype=Host  autostart=on  viewmode=Graphical redraw  formatstr='%15.6f'  grid=on  ylimits=[0,0]  nosamples=250  noprepostsamples=0  interleave=1  triggermode=FreeRun  triggersignal=1  trigsignalfromport=off  triggerlevel=0.0  triggerslope=Either  triggerscope=1  triggersample=0  filename=data.dat  mode=Lazy  writesize=512  autorestart=off  dynamicfilemode=off  maxwritefilesize=512*1024^2
  Selector72 : Selector  InputPortWidth=10  IndexOptions=Index vector (dialog)  Indices=[1,6]  OutputSizes=1
  Selector85 : Selector  InputPortWidth=20  IndexOptions=Index vector (dialog)  Indices=1  OutputSizes=1
  Selector86 : Selector  InputPortWidth=20  IndexOptions=Index vector (dialog)  Indices=2  OutputSizes=1
  Selector87 : Selector  InputPortWidth=20  IndexOptions=Index vector (dialog)  Indices=3  OutputSizes=1
  Selector88 : Selector  InputPortWidth=20  IndexOptions=Index vector (dialog)  Indices=1  OutputSizes=1
  Selector89 : Selector  InputPortWidth=20  IndexOptions=Index vector (dialog)  Indices=2  OutputSizes=1
  Selector90 : Selector  InputPortWidth=20  IndexOptions=Index vector (dialog)  Indices=3  OutputSizes=1
  Selector92 : Selector  InputPortWidth=10  IndexOptions=Index vector (dialog)  Indices=[2 7]  OutputSizes=1
  Selector94 : Selector  InputPortWidth=10  IndexOptions=Index vector (dialog)  Indices=[3 8]  OutputSizes=1
  Selector96 : Selector  InputPortWidth=10  IndexOptions=Index vector (dialog)  Indices=[4 9]  OutputSizes=1
  Selector98 : Selector  InputPortWidth=10  IndexOptions=Index vector (dialog)  Indices=[5 10]  OutputSizes=1
  wires:
  Bus Selector1/4 -> Mux3/2  "<Vy_tgd_des>"
  Bus Selector1/2 -> Mux2/2  "<Vx_tgd_des>"
  Gain7/1 -> Reshape6/1
  Gain8/1 -> Reshape5/1
  Gain9/1 -> Reshape4/1
  Gain10/1 -> Reshape1/1
  Bus Selector3/3 -> Gain8/1  "<ufp_sol_rel_com_x>"
  Bus Selector3/1 -> Gain10/1  "<ufp_sol_rel_st_x>"
  Bus Selector3/2 -> Gain9/1  "<ufp_sol_rel_st_y>"
  Bus Selector3/4 -> Gain7/1  "<ufp_sol_rel_com_y>"
  Gain3/1 -> Reshape3/1
  Gain2/1 -> Reshape2/1
  Mux3/1 -> Gain3/1
  Mux2/1 -> Gain2/1
  Bus Selector1/3 -> Mux3/1  "<vy_com_tgd>"
  Bus Selector1/1 -> Mux2/1  "<vx_com_tgd>"
  Selector85/1 -> Reshape47/1
  Selector90/1 -> Reshape52/1
  Bus Selector6/1 -> Gain16/1  "<q>"
  Bus Selector10/1 -> Gain11/1  "<rp_LToe>"
  Selector72/1 -> Reshape40/1
  Selector96/1 -> Reshape43/1
  Bus Selector9/1 -> Reshape73/1  "<Lx_stToe_stTD0_obs>"
  Bus Selector10/4 -> Gain14/1  "<rp_RToe_fil>"
  Selector98/1 -> Reshape44/1
  Gain11/1 -> Reshape79/1
  Selector94/1 -> Reshape42/1
  Selector92/1 -> Reshape41/1
  Selector87/1 -> Reshape49/1
  Bus Selector5/1 -> Selector98/1, Selector96/1, Selector94/1, Selector92/1, Selector72/1  "<u>"
  Bus Selector9/3 -> Reshape75/1  "<Lx_stToe_stTD0_kf>"
  Gain12/1 -> Reshape80/1
  Selector86/1 -> Reshape48/1
  Gain13/1 -> Reshape81/1
  Bus Selector6/2 -> Gain17/1  "<dq>"
  Gain17/1 -> Selector90/1, Selector89/1, Selector88/1
  Gain14/1 -> Reshape82/1
  Bus Selector10/2 -> Gain12/1  "<rp_RToe>"
  Bus Selector10/3 -> Gain13/1  "<rp_LToe_fil>"
  Selector89/1 -> Reshape51/1
  Bus Selector9/2 -> Reshape74/1  "<Ly_stToe_stTD0_obs>"
  Selector88/1 -> Reshape50/1
  Gain16/1 -> Selector86/1, Selector87/1, Selector85/1
  Bus Selector9/4 -> Reshape76/1  "<Ly_stToe_stTD0_kf>"
  In1/1 -> Bus Selector3/1, Bus Selector9/1, Bus Selector10/1, Bus Selector1/1, Bus Selector5/1, Bus Selector6/1
  Reshape47/1 -> Scope 1/1
  Reshape48/1 -> Scope 2/1
  Reshape49/1 -> Scope 3/1
  Reshape50/1 -> Scope 4/1
  Reshape51/1 -> Scope 5/1
  Reshape52/1 -> Scope 6/1
  Reshape40/1 -> Scope 7/1
  Reshape41/1 -> Scope 8/1
  Reshape42/1 -> Scope 9/1
  Reshape43/1 -> Scope 10/1
  Reshape44/1 -> Scope 11/1
  Reshape2/1 -> Scope 12/1
  Reshape3/1 -> Scope 13/1
  Reshape79/1 -> Scope 14/1
  Reshape80/1 -> Scope 15/1
  Reshape81/1 -> Scope 16/1
  Reshape82/1 -> Scope 17/1
  Reshape73/1 -> Scope 18/1
  Reshape74/1 -> Scope 19/1
  Reshape75/1 -> Scope 20/1
  Reshape76/1 -> Scope 21/1
  Reshape1/1 -> Scope 22/1
  Reshape4/1 -> Scope 23/1
  Reshape5/1 -> Scope 24/1
  Reshape6/1 -> Scope 25/1

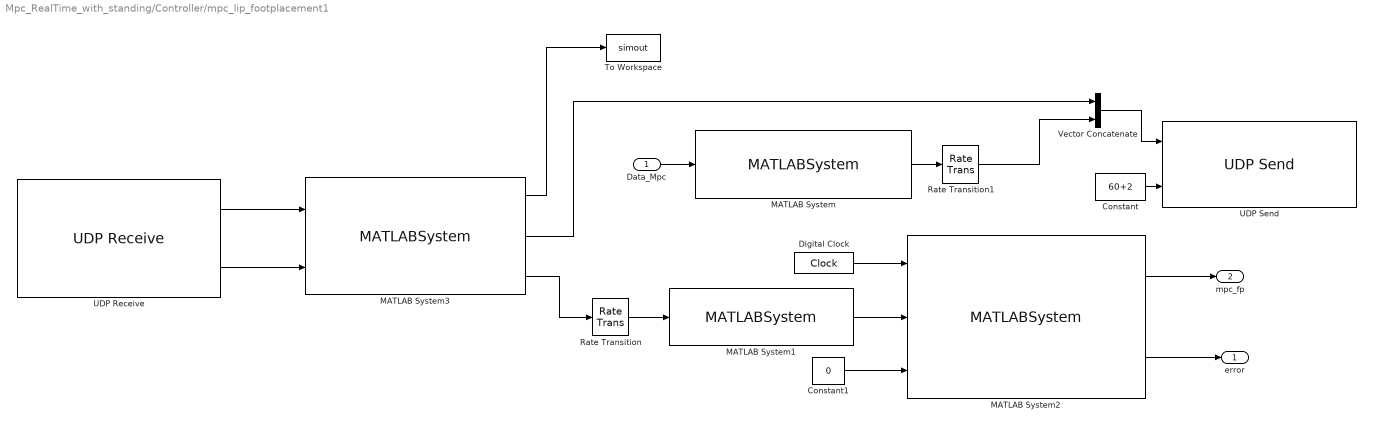
== system Mpc_RealTime_with_standing/Controller/mpc_lip_footplacement1 ==
  Data_Mpc : Inport
  Constant : Constant  Value=60+2
  Constant1 : Constant  Value=0
  Digital Clock : DigitalClock  SampleTime=sample_time
  MATLAB System : MATLABSystem  System=Pack_estimated_states  SimulateUsing=Code generation
      mask Type: Pack_estimated_states
      mask Display:
      | disp('Pack_estimated_states');
      | port_label('input',1,'Data_Mpc');
      | port_label('output',1,'bytes');
  MATLAB System1 : MATLABSystem  System=Unpack_mpc_lip_fp  SimulateUsing=Code generation
      mask Type: Unpack_mpc_lip_fp
      mask Display:
      | disp('Unpack_mpc_lip_fp');
      | port_label('input',1,'Data');
      | port_label('output',1,'data_bus');
  MATLAB System2 : MATLABSystem  System=udp_data_checker  SimulateUsing=Code generation
      mask Type: udp_data_checker
      mask Display:
      | disp('udp_data_checker');
      | port_label('input',1,'t');
      | port_label('input',2,'mpc_data_in');
      | port_label('input',3,'reset_error');
      | port_label('output',1,'mpc_data_out');
      | port_label('output',2,'err');
  MATLAB System3 : MATLABSystem  System=ProcessUdpPacket  heartbeatInterval=0.01  dataLength=20  SimulateUsing=Code generation
      mask Type: ProcessUdpPacket
      mask Display:
      | disp('ProcessUdpPacket');
      | port_label('input',1,'UDP Data');
      | port_label('input',2,'Length');
      | port_label('output',1,'Log');
      | port_label('output',2,'Header');
      | port_label('output',3,'Data');
  Rate Transition : RateTransition  InitialCondition=zeros(20,1)  OutPortSampleTime=sample_time
  Rate Transition1 : RateTransition  InitialCondition=zeros(60,1)  OutPortSampleTime=udp_sample_time
  To Workspace : ToWorkspace  VariableName=simout  SaveFormat=Timeseries  SampleTime=-1
  UDP Receive : xpcrtudplib/UDP Receive  ipAddressVal=Use host-target connection  localPort=27000  rcvWidth=20+2  rcvFmAny=off  fmAddress=10.10.10.150  maxUDPQueue=8  sampleTime=udp_sample_time
      settings: SourceProductName=Simulink Real-Time
  UDP Send : xpcrtudplib/UDP Send  ipAddressVal=Use host-target connection  localPort=27000  toAddress=10.10.10.150  toPort=28000  sampleTime=udp_sample_time
      settings: SourceProductName=Simulink Real-Time  SourceProductBaseCode=XP
  Vector Concatenate : Concatenate
  error : Outport
  mpc_fp : Outport  Port=2
  wires:
  Data_Mpc/1 -> MATLAB System/1
  MATLAB System3/3 -> Rate Transition/1
  Rate Transition/1 -> MATLAB System1/1
  MATLAB System1/1 -> MATLAB System2/2
  Rate Transition1/1 -> Vector Concatenate/2
  MATLAB System/1 -> Rate Transition1/1
  UDP Receive/2 -> MATLAB System3/2
  MATLAB System3/1 -> To Workspace/1
  MATLAB System3/2 -> Vector Concatenate/1
  Constant1/1 -> MATLAB System2/3
  Vector Concatenate/1 -> UDP Send/1
  MATLAB System2/2 -> error/1
  MATLAB System2/1 -> mpc_fp/1
  Digital Clock/1 -> MATLAB System2/1
  Constant/1 -> UDP Send/2
  UDP Receive/1 -> MATLAB System3/1

== matlab function Mpc_RealTime_with_standing/Controller/MATLAB Function1 ==
  data: dq input; dq output; dqxyz input; EulerRates input
function dq = mix_dq(dq,dqxyz,EulerRates)
dq(1:3) = dqxyz;
dq(4:6) = EulerRates;
